simulink model "parcial_ej3_20250609"  (R2021a)
settings: Solver=ode4  StartTime=0.0  StopTime=0.05  FixedStep=0.0001  RelTol=1e-3
libraries: cstblocks x1
settings Model: Creator=aghersin  LastModifiedBy=frand
settings SolverCC: AlgebraicLoopSolver=TrustRegion
settings DataIOCC: ReturnWorkspaceOutputs=off
settings OptimizationCC: LifeSpan=inf
settings DebuggingCC: SFExecutionAtInitializationDiag=none  SFMachineParentedDataDiag=warning  ArithmeticOperatorsInVariantConditions=warning
settings SFSimCC: SimUseLocalCustomCode=off  CustomCodeUndefinedFunction=UseInterfaceOnly
settings RTWCC: RTWUseLocalCustomCode=off
settings CodeAppCC: StateflowObjectComments=on

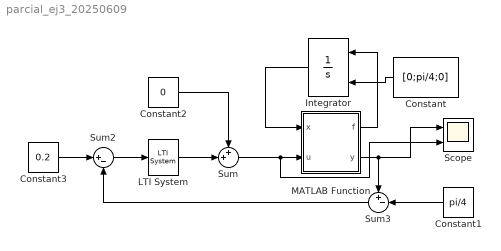
== system parcial_ej3_20250609 ==
  Constant : Constant  Value=[0;pi/4;0]
  Constant1 : Constant  Value=pi/4
  Constant2 : Constant  Value=0
  Constant3 : Constant  Value=0.2
  Integrator : Integrator  InitialConditionSource=external
  LTI System : cstblocks/LTI System  sys=C  IC=[]
  MATLAB Function : MATLAB Function  TreatAsAtomicUnit=on
  Scope : Scope  NumInputPorts=2
  Sum : Sum  Inputs=++|
  Sum2 : Sum  Inputs=|+-
  Sum3 : Sum  Inputs=+-|
  wires:
  Integrator/1 -> MATLAB Function/1(x)
  MATLAB Function/1(f) -> Integrator/1
  Constant/1 -> Integrator/2
  MATLAB Function/2(y) -> Sum3/1, Scope/1
  Constant1/1 -> Sum3/2
  Constant2/1 -> Sum/1
  Sum2/1 -> LTI System/1
  Constant3/1 -> Sum2/1
  Sum3/1 -> Sum2/2
  LTI System/1 -> Sum/2
  Sum/1 -> Scope/2, MATLAB Function/2(u)

== matlab function parcial_ej3_20250609/MATLAB Function ==
  data: x input; u input; f output; y output
function [f,y] = fcn(x,u)

alfa = 1.4595;
p=1000;

f1=-p*x(1)+p*u;
f2=x(3);
f3=-alfa*x(2)^3+sin(x(2))-x(3)+x(1);

f=[f1;f2;f3];

y=x(2);
